simulink model "eyetracker_bci_concept"  (R2024a)
settings: Solver=VariableStepAuto  StartTime=0.0  StopTime=inf  RelTol=1e-3
undefined symbols (not defined in the file): x, y
settings Model: Creator=Spencer  LastModifiedBy=Spencer

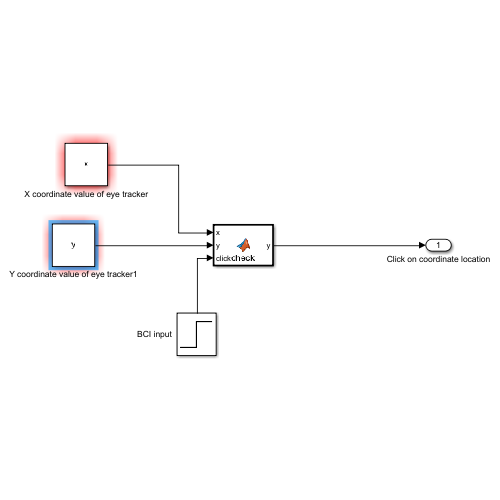
[thumbnail: Simulink's stored preview of the top-level diagram]
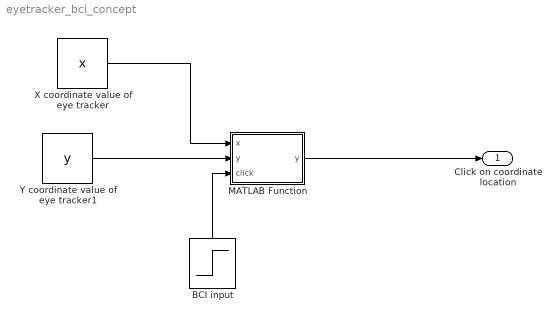
== system eyetracker_bci_concept ==
  BCI input : Step  SampleTime=0
  MATLAB Function : MATLAB Function  TreatAsAtomicUnit=on
  X coordinate value of eye tracker : Constant  Value=x
  Y coordinate value of eye tracker1 : Constant  Value=y
  Click on coordinate location : Outport
  wires:
  X coordinate value of eye tracker/1 -> MATLAB Function/1(x)
  BCI input/1 -> MATLAB Function/3(click)
  MATLAB Function/1(y) -> Click on coordinate location/1
  Y coordinate value of eye tracker1/1 -> MATLAB Function/2("y ")

== matlab function eyetracker_bci_concept/MATLAB Function ==
  data: x input; y input; y output; click input
function y = check(x,y,click)
%coord is 2x1 array: x is (1,1), y is (2,1)
%this function will check if click is true, if it is true it will click on
%the coordinate that the eye tracker is located
if click == 1
    y=[x y click];
else
    y=0;
